simulink library "mylib"  (R2020a)
settings: Solver=VariableStepAuto  StartTime=0.0  StopTime=10.0  RelTol=1e-3
undefined symbols (not defined in the file): d_du_max_pu, dir_to_bus1, dir_to_bus_0L, dir_to_bus_2, dir_to_line1, dir_to_line_0L, dir_to_line_2, du_max_pu, du_ph_max_pu, Fi_0, Fi_T_H, Fi_T_L, Fi_T_M, I0_calc_0L, I0_comp_H, I0_comp_L, I0_comp_M, I0_max_0L, I2_max_2, I_diff1, I_diff2, I_diff3, I_diff4, I_diff5, I_diff_to, I_hight_CT1_G, I_hight_CT2_G, I_low_CT1, I_low_CT2, I_max1, I_max2, I_max3, I_max4, I_max5, I_min_sec_CT1, I_min_sec_CT2, I_unb, Iph_max_0L, Iph_max_2, jmp_in_zone, jmp_in_zone_0L, jmp_in_zone_2, K_dop, max_min1, only_K1_0L, only_K1_2, only_K2_0L, only_K2_2, only_K3_0L, only_K3_2, P_ctl_0, PQ_Fi_ctl_0, Q_ctl_0, S_set_0, set, set1, T_fast, T_I_ctl, T_off, T_on ... (+15)
libraries: $bdroot x184, powerlib_meascontrol x97
(part 2 of 14)

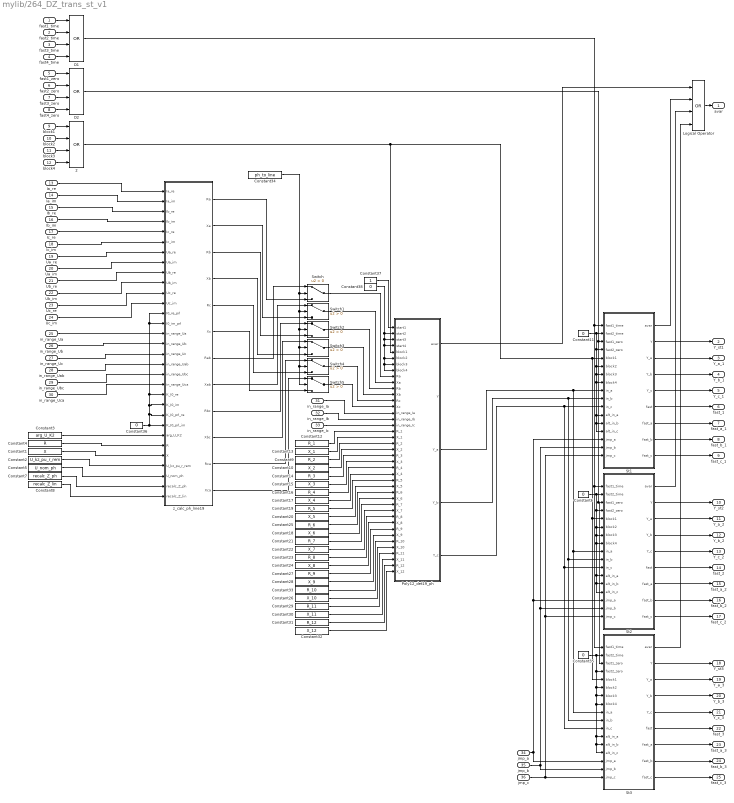
== system mylib/264_DZ_trans_st_v1 ==
  fast1_time : Inport
  fast2_time : Inport  Port=2
  fast3_time : Inport  Port=3
  fast4_time : Inport  Port=4
  fast1_zero : Inport  Port=5
  fast2_zero : Inport  Port=6
  fast3_zero : Inport  Port=7
  fast4_zero : Inport  Port=8
  block1 : Inport  Port=9
  block2 : Inport  Port=10
  block3 : Inport  Port=11
  block4 : Inport  Port=12
  Ia_re : Inport  Port=13
  Ia_im : Inport  Port=14
  Ib_re : Inport  Port=15
  Ib_im : Inport  Port=16
  Ic_re : Inport  Port=17
  Ic_im : Inport  Port=18
  Ua_re : Inport  Port=19
  Ua_im : Inport  Port=20
  Ub_re : Inport  Port=21
  Ub_im : Inport  Port=22
  Uc_re : Inport  Port=23
  Uc_im : Inport  Port=24
  in_range_Ua : Inport  Port=25
  in_range_Ub : Inport  Port=26
  in_range_Uc : Inport  Port=27
  in_range_Uab : Inport  Port=28
  in_range_Ubc : Inport  Port=29
  in_range_Uca : Inport  Port=30
  in_range_Ia : Inport  Port=31
  in_range_Ib : Inport  Port=32
  in_range_Ic : Inport  Port=33
  jmp_a : Inport  Port=34
  jmp_b : Inport  Port=35
  jmp_c : Inport  Port=36
  2 : Logic  Operator=OR  Inputs=4  AllPortsSameDT=off  OutDataTypeStr=boolean
  Constant1 : Constant  Value=X
  Constant10 : Constant  Value=X_2
  Constant{6,11,35..36,38} (5 alike) : Constant  Value=0
  Constant12 : Constant  Value=R_1
  Constant13 : Constant  Value=X_1
  Constant14 : Constant  Value=R_3
  Constant15 : Constant  Value=X_3
  Constant16 : Constant  Value=R_4
  Constant17 : Constant  Value=X_4
  Constant18 : Constant  Value=X_6
  Constant19 : Constant  Value=R_5
  Constant2 : Constant  Value=U_kz_pu_r_rem
  Constant20 : Constant  Value=X_5
  Constant21 : Constant  Value=R_7
  Constant22 : Constant  Value=X_7
  Constant23 : Constant  Value=R_8
  Constant24 : Constant  Value=X_8
  Constant25 : Constant  Value=R_6
  Constant26 : Constant  Value=X_10
  Constant27 : Constant  Value=R_9
  Constant28 : Constant  Value=X_9
  Constant29 : Constant  Value=R_11
  Constant3 : Constant  Value=arg_U_K2
  Constant30 : Constant  Value=X_11
  Constant31 : Constant  Value=R_12
  Constant32 : Constant  Value=X_12
  Constant33 : Constant  Value=R_10
  Constant34 : Constant  Value=ph_to_line
  Constant37 : Constant
  Constant4 : Constant  Value=R
  Constant5 : Constant  Value=U_nom_ph
  Constant7 : Constant  Value=recalc_Z_ph
  Constant8 : Constant  Value=recalc_Z_lin
  Constant9 : Constant  Value=R_2
  D1 : Logic  Operator=OR  Inputs=4  AllPortsSameDT=off  OutDataTypeStr=boolean
  D2 : Logic  Operator=OR  Inputs=4  AllPortsSameDT=off  OutDataTypeStr=boolean
  Logical Operator : Logic  Operator=OR  Inputs=4  AllPortsSameDT=off  OutDataTypeStr=boolean
  Poly12_det19_ph : Subsystem
  St1 : Subsystem  AncestorBlock=mylib/230_st18_ph  mask{st18_ph=[1, 1, 1, jmp_in_zone, T_reset, T_fast, T_st1, T_out]}
      mask prompts: st18_ph "st18_ph [only_K1, only_K2, only_K3, jmp_in_zone, T_reset, T_fast, T_st, T_out]"
      mask init:
      | only_K1 = st18_ph(1);
      | only_K2 = st18_ph(2); 
      | only_K3 = st18_ph(3); 
      | jmp_in_zone = st18_ph(4);
      | T_reset = st18_ph(5);
      | T_fast = st18_ph(6); 
      | T_st = st18_ph(7); 
      | T_out = st18_ph(8);
  St2 : Subsystem  AncestorBlock=mylib/230_st18_ph  mask{st18_ph=[1, 1, 1, jmp_in_zone, T_reset, T_fast, T_st2, T_out]}
      mask prompts: st18_ph "st18_ph [only_K1, only_K2, only_K3, jmp_in_zone, T_reset, T_fast, T_st, T_out]"
      mask init:
      | only_K1 = st18_ph(1);
      | only_K2 = st18_ph(2); 
      | only_K3 = st18_ph(3); 
      | jmp_in_zone = st18_ph(4);
      | T_reset = st18_ph(5);
      | T_fast = st18_ph(6); 
      | T_st = st18_ph(7); 
      | T_out = st18_ph(8);
  St3 : Subsystem  AncestorBlock=mylib/230_st18_ph  mask{st18_ph=[1, 1, 1, jmp_in_zone, T_reset, T_fast, T_st3, T_out]}
      mask prompts: st18_ph "st18_ph [only_K1, only_K2, only_K3, jmp_in_zone, T_reset, T_fast, T_st, T_out]"
      mask init:
      | only_K1 = st18_ph(1);
      | only_K2 = st18_ph(2); 
      | only_K3 = st18_ph(3); 
      | jmp_in_zone = st18_ph(4);
      | T_reset = st18_ph(5);
      | T_fast = st18_ph(6); 
      | T_st = st18_ph(7); 
      | T_out = st18_ph(8);
  Switch{,1..5} (6 alike) : Switch  Criteria=u2 > Threshold
  z_calc_ph_line19 : Subsystem
  avar : Outport
  Y_st1 : Outport  Port=2
  Y_a_1 : Outport  Port=3
  Y_b_1 : Outport  Port=4
  Y_c_1 : Outport  Port=5
  fast_1 : Outport  Port=6
  fast_a_1 : Outport  Port=7
  fast_b_1 : Outport  Port=8
  fast_c_1 : Outport  Port=9
  Y_st2 : Outport  Port=10
  Y_a_2 : Outport  Port=11
  Y_b_2 : Outport  Port=12
  Y_c_2 : Outport  Port=13
  fast_2 : Outport  Port=14
  fast_a_2 : Outport  Port=15
  fast_b_2 : Outport  Port=16
  fast_c_2 : Outport  Port=17
  Y_st3 : Outport  Port=18
  Y_a_3 : Outport  Port=19
  Y_b_3 : Outport  Port=20
  Y_c_3 : Outport  Port=21
  fast_3 : Outport  Port=22
  fast_a_3 : Outport  Port=23
  fast_b_3 : Outport  Port=24
  fast_c_3 : Outport  Port=25
  wires:
  block4/1 -> 2/4
  block3/1 -> 2/3
  block2/1 -> 2/2
  block1/1 -> 2/1
  fast2_time/1 -> D1/2
  fast4_time/1 -> D1/4
  fast3_time/1 -> D1/3
  fast1_time/1 -> D1/1
  St1/2(Y) -> Y_st1/1
  Constant11/1 -> St1/2(fast2_time), St1/14(alt_in_c), St1/13(alt_in_b), St1/12(alt_in_a), St1/8(block4), St1/7(block3), St1/6(block2), St1/4(fast2_zero)
  Logical Operator/1 -> avar/1
  Constant6/1 -> St2/2(fast2_time), St2/14(alt_in_c), St2/13(alt_in_b), St2/12(alt_in_a), St2/8(block4), St2/7(block3), St2/6(block2), St2/4(fast2_zero)
  jmp_a/1 -> St3/15(jmp_a), St1/15(jmp_a), St2/15(jmp_a)
  jmp_c/1 -> St3/17(jmp_c), St1/17(jmp_c), St2/17(jmp_c)
  jmp_b/1 -> St3/16(jmp_b), St1/16(jmp_b), St2/16(jmp_b)
  St2/2(Y) -> Y_st2/1
  St1/1(avar) -> Logical Operator/2
  St2/1(avar) -> Logical Operator/3
  fast3_zero/1 -> D2/3
  fast2_zero/1 -> D2/2
  fast1_zero/1 -> D2/1
  fast4_zero/1 -> D2/4
  Constant35/1 -> St3/2(fast2_time), St3/14(alt_in_c), St3/13(alt_in_b), St3/12(alt_in_a), St3/8(block4), St3/7(block3), St3/6(block2), St3/4(fast2_zero)
  Constant36/1 -> z_calc_ph_line19/23(K_I0_prl_re), z_calc_ph_line19/22(K_I0_im), z_calc_ph_line19/13(I0_re_prl), z_calc_ph_line19/14(I0_im_prl), z_calc_ph_line19/21(K_I0_re), z_calc_ph_line19/24(K_I0_prl_im)
  Ia_re/1 -> z_calc_ph_line19/1(Ia_re)
  Ia_im/1 -> z_calc_ph_line19/2(Ia_im)
  Ib_re/1 -> z_calc_ph_line19/3(Ib_re)
  Ib_im/1 -> z_calc_ph_line19/4(Ib_im)
  Ic_re/1 -> z_calc_ph_line19/5(Ic_re)
  Ic_im/1 -> z_calc_ph_line19/6(Ic_im)
  Ua_re/1 -> z_calc_ph_line19/7(Ua_re)
  Ua_im/1 -> z_calc_ph_line19/8(Ua_im)
  Ub_re/1 -> z_calc_ph_line19/9(Ub_re)
  Ub_im/1 -> z_calc_ph_line19/10(Ub_im)
  Uc_re/1 -> z_calc_ph_line19/11(Uc_re)
  Uc_im/1 -> z_calc_ph_line19/12(Uc_im)
  in_range_Ua/1 -> z_calc_ph_line19/15(in_range_Ua)
  in_range_Ub/1 -> z_calc_ph_line19/16(in_range_Ub)
  in_range_Uc/1 -> z_calc_ph_line19/17(in_range_Uc)
  in_range_Uab/1 -> z_calc_ph_line19/18(in_range_Uab)
  in_range_Ubc/1 -> z_calc_ph_line19/19(in_range_Ubc)
  in_range_Uca/1 -> z_calc_ph_line19/20(in_range_Uca)
  Constant3/1 -> z_calc_ph_line19/25(arg_U_K2)
  Constant4/1 -> z_calc_ph_line19/26(R)
  Constant8/1 -> z_calc_ph_line19/31(recalc_Z_lin)
  Constant7/1 -> z_calc_ph_line19/30(recalc_Z_ph)
  Constant5/1 -> z_calc_ph_line19/29(U_nom_ph)
  Constant2/1 -> z_calc_ph_line19/28(U_kz_pu_r_rem)
  Constant1/1 -> z_calc_ph_line19/27(X)
  Constant12/1 -> Poly12_det19_ph/18(R_1)
  Constant13/1 -> Poly12_det19_ph/19(X_1)
  Constant9/1 -> Poly12_det19_ph/20(R_2)
  Constant10/1 -> Poly12_det19_ph/21(X_2)
  Constant32/1 -> Poly12_det19_ph/41(X_12)
  Constant31/1 -> Poly12_det19_ph/40(R_12)
  Constant30/1 -> Poly12_det19_ph/39(X_11)
  Constant29/1 -> Poly12_det19_ph/38(R_11)
  Constant26/1 -> Poly12_det19_ph/37(X_10)
  Constant33/1 -> Poly12_det19_ph/36(R_10)
  Constant28/1 -> Poly12_det19_ph/35(X_9)
  Constant27/1 -> Poly12_det19_ph/34(R_9)
  Constant24/1 -> Poly12_det19_ph/33(X_8)
  Constant23/1 -> Poly12_det19_ph/32(R_8)
  Constant22/1 -> Poly12_det19_ph/31(X_7)
  Constant21/1 -> Poly12_det19_ph/30(R_7)
  Constant18/1 -> Poly12_det19_ph/29(X_6)
  Constant25/1 -> Poly12_det19_ph/28(R_6)
  Constant20/1 -> Poly12_det19_ph/27(X_5)
  Constant19/1 -> Poly12_det19_ph/26(R_5)
  Constant17/1 -> Poly12_det19_ph/25(X_4)
  Constant16/1 -> Poly12_det19_ph/24(R_4)
  Constant15/1 -> Poly12_det19_ph/23(X_3)
  Constant14/1 -> Poly12_det19_ph/22(R_3)
  Constant34/1 -> Switch5/2, Switch4/2, Switch3/2, Switch2/2, Switch1/2, Switch/2
  z_calc_ph_line19/7(Rab) -> Switch/1
  z_calc_ph_line19/8(Xab) -> Switch1/1
  z_calc_ph_line19/9(Rbc) -> Switch2/1
  z_calc_ph_line19/10(Xbc) -> Switch3/1
  z_calc_ph_line19/11(Rca) -> Switch4/1
  z_calc_ph_line19/12(Xca) -> Switch5/1
  z_calc_ph_line19/6(Xc) -> Switch5/3
  z_calc_ph_line19/5(Rc) -> Switch4/3
  z_calc_ph_line19/4(Xb) -> Switch3/3
  z_calc_ph_line19/3(Rb) -> Switch2/3
  z_calc_ph_line19/2(Xa) -> Switch1/3
  z_calc_ph_line19/1(Ra) -> Switch/3
  Switch5/1 -> Poly12_det19_ph/14(Xc)
  Switch4/1 -> Poly12_det19_ph/13(Rc)
  Switch3/1 -> Poly12_det19_ph/12(Xb)
  Switch2/1 -> Poly12_det19_ph/11(Rb)
  Switch1/1 -> Poly12_det19_ph/10(Xa)
  Switch/1 -> Poly12_det19_ph/9(Ra)
  in_range_Ic/1 -> Poly12_det19_ph/17(in_range_Ic)
  in_range_Ib/1 -> Poly12_det19_ph/16(in_range_Ib)
  in_range_Ia/1 -> Poly12_det19_ph/15(in_range_Ia)
  Poly12_det19_ph/3(Y_a) -> St3/9(in_a), St2/9(in_a), St1/9(in_a)
  Poly12_det19_ph/4(Y_b) -> St3/10(in_b), St2/10(in_b), St1/10(in_b)
  Poly12_det19_ph/5(Y_c) -> St3/11(in_c), St2/11(in_c), St1/11(in_c)
  St3/2(Y) -> Y_st3/1
  Poly12_det19_ph/1(avar) -> Logical Operator/1
  St3/1(avar) -> Logical Operator/4
  St1/3(Y_a) -> Y_a_1/1
  St1/4(Y_b) -> Y_b_1/1
  St1/5(Y_c) -> Y_c_1/1
  St1/6(fast) -> fast_1/1
  St1/7(fast_a) -> fast_a_1/1
  St1/9(fast_c) -> fast_c_1/1
  St1/8(fast_b) -> fast_b_1/1
  St2/3(Y_a) -> Y_a_2/1
  St2/4(Y_b) -> Y_b_2/1
  St2/5(Y_c) -> Y_c_2/1
  St2/6(fast) -> fast_2/1
  St2/7(fast_a) -> fast_a_2/1
  St2/8(fast_b) -> fast_b_2/1
  St2/9(fast_c) -> fast_c_2/1
  St3/9(fast_c) -> fast_c_3/1
  St3/8(fast_b) -> fast_b_3/1
  St3/7(fast_a) -> fast_a_3/1
  St3/6(fast) -> fast_3/1
  St3/5(Y_c) -> Y_c_3/1
  St3/4(Y_b) -> Y_b_3/1
  St3/3(Y_a) -> Y_a_3/1
  2/1 -> Poly12_det19_ph/5(block1), St3/5(block1), St2/5(block1), St1/5(block1)
  Constant37/1 -> Poly12_det19_ph/1(start1)
  Constant38/1 -> Poly12_det19_ph/8(block4), Poly12_det19_ph/7(block3), Poly12_det19_ph/6(block2), Poly12_det19_ph/4(start4), Poly12_det19_ph/3(start3), Poly12_det19_ph/2(start2)
  D2/1 -> St3/3(fast1_zero), St2/3(fast1_zero), St1/3(fast1_zero)
  D1/1 -> St3/1(fast1_time), St2/1(fast1_time), St1/1(fast1_time)

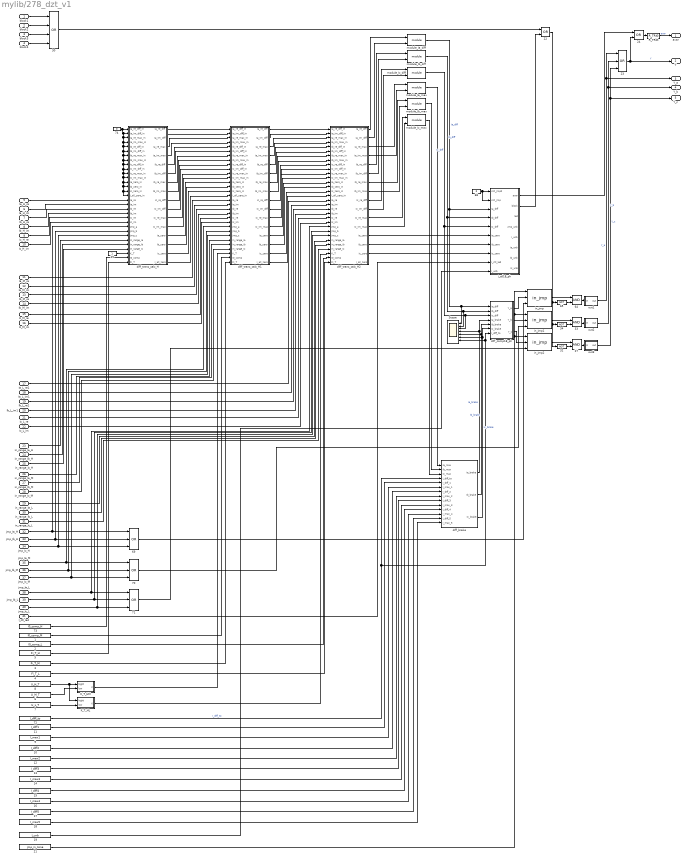
== system mylib/278_dzt_v1 ==
  block1 : Inport
  block2 : Inport  Port=2
  block3 : Inport  Port=3
  block4 : Inport  Port=4
  Ia_H_re : Inport  Port=5
  Ia_H_im : Inport  Port=6
  Ib_H_re : Inport  Port=7
  Ib_H_im : Inport  Port=8
  Ic_H_re : Inport  Port=9
  Ic_H_im : Inport  Port=10
  Ia_M_re : Inport  Port=11
  Ia_M_im : Inport  Port=12
  Ib_M_re : Inport  Port=13
  Ib_M_im : Inport  Port=14
  Ic_M_re : Inport  Port=15
  Ic_M_im : Inport  Port=16
  Ia_L_re1 : Inport  Port=17
  Ia_L_im1 : Inport  Port=18
  Ib_L_re1 : Inport  Port=19
  Ib_L_im1 : Inport  Port=20
  Ic_L_re : Inport  Port=21
  Ic_L_im : Inport  Port=22
  in_range_Ia_H : Inport  Port=23
  in_range_Ib_H : Inport  Port=24
  in_range_Ic_H : Inport  Port=25
  in_range_Ia_M : Inport  Port=26
  in_range_Ib_M : Inport  Port=27
  in_range_Ic_M : Inport  Port=28
  in_range_Ia_L : Inport  Port=29
  in_range_Ib_L : Inport  Port=30
  in_range_Ic_L : Inport  Port=31
  jmp_Ia_H : Inport  Port=32
  jmp_Ib_H : Inport  Port=33
  jmp_Ic_H : Inport  Port=34
  jmp_Ia_M : Inport  Port=35
  jmp_Ib_M : Inport  Port=36
  jmp_Ic_M : Inport  Port=37
  jmp_Ia_L : Inport  Port=38
  jmp_Ib_L : Inport  Port=39
  jmp_Ic_L : Inport  Port=40
  I_ctl_led : Inport  Port=41
  1 : Constant  Value=I0_comp_M
  10 : Constant  Value=I_diff2
  11 : Constant  Value=I_diff1
  12 : Constant  Value=I_max2
  13 : Constant  Value=I_diff3
  14 : Constant  Value=I_max3
  15 : Constant  Value=I_diff4
  16 : Constant  Value=I_max4
  17 : Constant  Value=I_diff5
  18 : Constant  Value=I_max5
  19 : Constant  Value=I_unb
  2 : Constant  Value=I0_comp_L
  21 : Constant  Value=jmp_in_zone
  22 : Logic  Operator=OR  AllPortsSameDT=off  OutDataTypeStr=boolean
  {23,69..71} (4 alike) : Logic  Operator=OR  Inputs=3  AllPortsSameDT=off  OutDataTypeStr=boolean
  24 : Logic  Operator=OR  AllPortsSameDT=off  OutDataTypeStr=boolean
  25 : Constant
  27 : Logic  AllPortsSameDT=off  OutDataTypeStr=boolean
  3 : Constant  Value=Fi_T_M
  30 : Logic  Operator=OR  Inputs=4  AllPortsSameDT=off  OutDataTypeStr=boolean
  32 : Logic  Operator=NOT  AllPortsSameDT=off  OutDataTypeStr=boolean
  33 : Logic  AllPortsSameDT=off  OutDataTypeStr=boolean
  34 : Logic  Operator=NOT  AllPortsSameDT=off  OutDataTypeStr=boolean
  4 : Constant  Value=Fi_T_L
  5 : Constant  Value=Fi_T_H
  6 : Constant  Value=U_M_T
  64 : Logic  AllPortsSameDT=off  OutDataTypeStr=boolean
  65 : Logic  Operator=NOT  AllPortsSameDT=off  OutDataTypeStr=boolean
  68 : Constant  Value=0
  7 : Constant  Value=U_L_T
  72 : Constant  Value=I_diff_to
  73 : Constant  Value=I0_comp_H
  74 : Constant  Value=0
  8 : Constant  Value=U_H_T
  9 : Constant  Value=I_max1
  K_T_HL : Subsystem
  K_T_HM : Subsystem
  R_TRIG : $bdroot/R_TRIG  SystemSampleTime=-1  Latency=0  AutoFrameSizeCalculation=off
  Scope : Scope  NumInputPorts=7
  diff_brake : Subsystem
  diff_comp18_ph : Subsystem
  diff_trans_calc_H : Subsystem
  diff_trans_calc_H1 : Subsystem
  diff_trans_calc_H2 : Subsystem
  i_ctl18_ph : Subsystem  mask{CTL=[T_I_ctl]}
      mask prompts: CTL "CTL[T_I_ctl]"
      mask init:
      | T_I_ctl = CTL(1);
  in_jmp : $bdroot/in_jmp  in_jmp=[T_reset]
  in_jmp1 : $bdroot/in_jmp  in_jmp=[T_reset]
  in_jmp2 : $bdroot/in_jmp  in_jmp=[T_reset]
  module_Ia_diff : $bdroot/module  SystemSampleTime=-1  Latency=0  AutoFrameSizeCalculation=off
  module_Ia_max : $bdroot/module  SystemSampleTime=-1  Latency=0  AutoFrameSizeCalculation=off
  module_Ib_diff : $bdroot/module  SystemSampleTime=-1  Latency=0  AutoFrameSizeCalculation=off
  module_Ib_max : $bdroot/module  SystemSampleTime=-1  Latency=0  AutoFrameSizeCalculation=off
  module_Ic_diff : $bdroot/module  SystemSampleTime=-1  Latency=0  AutoFrameSizeCalculation=off
  module_Ic_max : $bdroot/module  SystemSampleTime=-1  Latency=0  AutoFrameSizeCalculation=off
  out1 : Subsystem  mask{out=[T_out]}
      mask prompts: out "out[T_out]"
      mask init:
      | T_out = out(1);
  out2 : Subsystem  mask{out=[T_out]}
      mask prompts: out "out[T_out]"
      mask init:
      | T_out = out(1);
  out3 : Subsystem  mask{out=[T_out]}
      mask prompts: out "out[T_out]"
      mask init:
      | T_out = out(1);
  avar : Outport
  Y : Outport  Port=2
  Y_a : Outport  Port=3
  Y_b : Outport  Port=4
  Y_c : Outport  Port=5
  wires:
  I_ctl_led/1 -> i_ctl18_ph/9(I_ctl_led)
  22/1 -> 65/1, 34/1, 32/1
  R_TRIG/1 -> avar/1  "avar"
  out3/1(out) -> 23/3, Y_c/1  "Y_c"
  out2/1(out) -> 23/2, Y_b/1  "Y_b"
  out1/1(out) -> 23/1, Y_a/1  "Y_a"
  i_ctl18_ph/1(avar) -> 24/1
  24/1 -> R_TRIG/1
  23/1 -> Y/1, 24/2  "Y"
  30/1 -> 22/1
  i_ctl18_ph/2(block) -> 22/2
  65/1 -> 64/2
  34/1 -> 33/2
  in_range_Ib_M/1 -> diff_trans_calc_H1/27(in_range_Ib)
  jmp_Ic_L/1 -> 71/3, diff_trans_calc_H2/25(jmp_c)
  in_range_Ic_L/1 -> diff_trans_calc_H2/28(in_range_Ic)
  jmp_Ia_L/1 -> 71/1, diff_trans_calc_H2/23(jmp_a)
  jmp_Ib_M/1 -> 70/2, diff_trans_calc_H1/24(jmp_b)
  jmp_Ia_M/1 -> 70/1, diff_trans_calc_H1/23(jmp_a)
  jmp_Ib_H/1 -> 69/2, diff_trans_calc_H/24(jmp_b)
  jmp_Ic_H/1 -> 69/3, diff_trans_calc_H/25(jmp_c)
  in_range_Ib_H/1 -> diff_trans_calc_H/27(in_range_Ib)
  in_range_Ic_H/1 -> diff_trans_calc_H/28(in_range_Ic)
  in_range_Ia_L/1 -> diff_trans_calc_H2/26(in_range_Ia)
  jmp_Ia_H/1 -> diff_trans_calc_H/23(jmp_a), 69/1
  74/1 -> diff_trans_calc_H/1(Ia_re_diff_in), diff_trans_calc_H/2(Ia_im_diff_in), diff_trans_calc_H/16(I_all_zero_in), diff_trans_calc_H/15(Ic_zero_in), diff_trans_calc_H/14(Ib_zero_in), diff_trans_calc_H/13(Ia_zero_in), diff_trans_calc_H/12(Ic_im_max_in), diff_trans_calc_H/11(Ic_re_max_in), diff_trans_calc_H/10(Ic_im_diff_in), diff_trans_calc_H/9(Ic_re_diff_in), diff_trans_calc_H/8(Ib_im_max_in), diff_trans_calc_H/7(Ib_re_max_in), diff_trans_calc_H/6(Ib_im_diff_in), diff_trans_calc_H/5(Ib_re_diff_in), diff_trans_calc_H/4(Ia_im_max_in), diff_trans_calc_H/3(Ia_re_max_in)
  73/1 -> diff_trans_calc_H/30(I0_comp)
  Ic_L_re/1 -> diff_trans_calc_H2/21(Ic_re)
  Ib_L_im1/1 -> diff_trans_calc_H2/20(Ib_im)
  Ib_L_re1/1 -> diff_trans_calc_H2/19(Ib_re)
  Ia_L_im1/1 -> diff_trans_calc_H2/18(Ia_im)
  Ic_L_im/1 -> diff_trans_calc_H2/22(Ic_im)
  Ia_L_re1/1 -> diff_trans_calc_H2/17(Ia_re)
  diff_trans_calc_H1/2(Ia_im_diff) -> diff_trans_calc_H2/2(Ia_im_diff_in)
  diff_trans_calc_H1/3(Ia_re_max) -> diff_trans_calc_H2/3(Ia_re_max_in)
  diff_trans_calc_H1/4(Ia_im_max) -> diff_trans_calc_H2/4(Ia_im_max_in)
  diff_trans_calc_H1/5(Ib_re_diff) -> diff_trans_calc_H2/5(Ib_re_diff_in)
  diff_trans_calc_H1/6(Ib_im_diff) -> diff_trans_calc_H2/6(Ib_im_diff_in)
  diff_trans_calc_H1/7(Ib_re_max) -> diff_trans_calc_H2/7(Ib_re_max_in)
  diff_trans_calc_H1/8(Ib_im_max) -> diff_trans_calc_H2/8(Ib_im_max_in)
  diff_trans_calc_H1/9(Ic_re_diff) -> diff_trans_calc_H2/9(Ic_re_diff_in)
  diff_trans_calc_H1/10(Ic_im_diff) -> diff_trans_calc_H2/10(Ic_im_diff_in)
  diff_trans_calc_H1/11(Ic_re_max) -> diff_trans_calc_H2/11(Ic_re_max_in)
  diff_trans_calc_H1/12(Ic_im_max) -> diff_trans_calc_H2/12(Ic_im_max_in)
  diff_trans_calc_H1/13(Ia_zero) -> diff_trans_calc_H2/13(Ia_zero_in)
  diff_trans_calc_H1/14(Ib_zero) -> diff_trans_calc_H2/14(Ib_zero_in)
  diff_trans_calc_H1/15(Ic_zero) -> diff_trans_calc_H2/15(Ic_zero_in)
  2/1 -> diff_trans_calc_H2/30(I0_comp)
  4/1 -> diff_trans_calc_H2/31(Fi_T)
  K_T_HL/1(K) -> diff_trans_calc_H2/29(K_T)
  K_T_HM/1(K) -> diff_trans_calc_H1/29(K_T)
  3/1 -> diff_trans_calc_H1/31(Fi_T)
  diff_trans_calc_H/2(Ia_im_diff) -> diff_trans_calc_H1/2(Ia_im_diff_in)
  diff_trans_calc_H/3(Ia_re_max) -> diff_trans_calc_H1/3(Ia_re_max_in)
  diff_trans_calc_H/4(Ia_im_max) -> diff_trans_calc_H1/4(Ia_im_max_in)
  diff_trans_calc_H/5(Ib_re_diff) -> diff_trans_calc_H1/5(Ib_re_diff_in)
  diff_trans_calc_H/6(Ib_im_diff) -> diff_trans_calc_H1/6(Ib_im_diff_in)
  diff_trans_calc_H/7(Ib_re_max) -> diff_trans_calc_H1/7(Ib_re_max_in)
  diff_trans_calc_H/8(Ib_im_max) -> diff_trans_calc_H1/8(Ib_im_max_in)
  diff_trans_calc_H/9(Ic_re_diff) -> diff_trans_calc_H1/9(Ic_re_diff_in)
  diff_trans_calc_H/10(Ic_im_diff) -> diff_trans_calc_H1/10(Ic_im_diff_in)
  diff_trans_calc_H/11(Ic_re_max) -> diff_trans_calc_H1/11(Ic_re_max_in)
  diff_trans_calc_H/12(Ic_im_max) -> diff_trans_calc_H1/12(Ic_im_max_in)
  diff_trans_calc_H/13(Ia_zero) -> diff_trans_calc_H1/13(Ia_zero_in)
  diff_trans_calc_H/14(Ib_zero) -> diff_trans_calc_H1/14(Ib_zero_in)
  diff_trans_calc_H/15(Ic_zero) -> diff_trans_calc_H1/15(Ic_zero_in)
  Ib_M_re/1 -> diff_trans_calc_H1/19(Ib_re)
  Ib_M_im/1 -> diff_trans_calc_H1/20(Ib_im)
  Ic_M_re/1 -> diff_trans_calc_H1/21(Ic_re)
  Ic_M_im/1 -> diff_trans_calc_H1/22(Ic_im)
  Ia_M_im/1 -> diff_trans_calc_H1/18(Ia_im)
  Ia_M_re/1 -> diff_trans_calc_H1/17(Ia_re)
  Ic_H_re/1 -> diff_trans_calc_H/21(Ic_re)
  Ic_H_im/1 -> diff_trans_calc_H/22(Ic_im)
  Ib_H_im/1 -> diff_trans_calc_H/20(Ib_im)
  Ib_H_re/1 -> diff_trans_calc_H/19(Ib_re)
  Ia_H_im/1 -> diff_trans_calc_H/18(Ia_im)
  Ia_H_re/1 -> diff_trans_calc_H/17(Ia_re)
  module_Ic_max/1 -> diff_brake/3(Ic_max)
  module_Ib_max/1 -> diff_brake/2(Ib_max)
  module_Ia_max/1 -> diff_brake/1(Ia_max)
  18/1 -> diff_brake/14(I_max_5)
  17/1 -> diff_brake/13(I_diff_5)
  16/1 -> diff_brake/12(I_max_4)
  15/1 -> diff_brake/11(I_diff_4)
  14/1 -> diff_brake/10(I_max_3)
  13/1 -> diff_brake/9(I_diff_3)
  12/1 -> diff_brake/8(I_max_2)
  10/1 -> diff_brake/7(I_diff_2)
  9/1 -> diff_brake/6(I_max_1)
  11/1 -> diff_brake/5(I_diff_1)
  72/1 -> diff_comp18_ph/7(I_diff_to), Scope/7, diff_brake/4(I_diff_to)  "I_diff_to"
  69/1 -> in_jmp/3
  70/1 -> in_jmp1/3
  71/1 -> in_jmp2/3
  jmp_Ic_M/1 -> 70/3, diff_trans_calc_H1/25(jmp_c)
  jmp_Ib_L/1 -> 71/2, diff_trans_calc_H2/24(jmp_b)
  21/1 -> in_jmp/1, in_jmp1/1, in_jmp2/1
  module_Ib_diff/1 -> i_ctl18_ph/4(Ib_diff), diff_comp18_ph/2(Ib_diff), Scope/2  "Ib_diff"
  68/1 -> i_ctl18_ph/1(cnt_jmp0), i_ctl18_ph/2(cnt_jmp)
  diff_trans_calc_H2/15(Ic_zero) -> i_ctl18_ph/8(Ic_zero)
  diff_trans_calc_H2/14(Ib_zero) -> i_ctl18_ph/7(Ib_zero)
  diff_trans_calc_H2/13(Ia_zero) -> i_ctl18_ph/6(Ia_zero)
  module_Ia_diff/1 -> i_ctl18_ph/3(Ia_diff), diff_comp18_ph/1(Ia_diff), Scope/1  "Ia_diff"
  module_Ic_diff/1 -> i_ctl18_ph/5(Ic_diff), diff_comp18_ph/3(Ic_diff), Scope/3  "Ic_diff"
  diff_comp18_ph/1(Y_a) -> in_jmp/2
  diff_comp18_ph/2(Y_b) -> in_jmp1/2
  diff_comp18_ph/3(Y_c) -> in_jmp2/2
  diff_trans_calc_H2/1(Ia_re_diff) -> module_Ia_diff/1
  diff_trans_calc_H2/2(Ia_im_diff) -> module_Ia_diff/2
  diff_trans_calc_H2/9(Ic_re_diff) -> module_Ic_diff/1
  diff_trans_calc_H2/3(Ia_re_max) -> module_Ia_max/1
  diff_trans_calc_H2/4(Ia_im_max) -> module_Ia_max/2
  diff_trans_calc_H2/10(Ic_im_diff) -> module_Ic_diff/2
  diff_trans_calc_H2/5(Ib_re_diff) -> module_Ib_diff/1
  diff_trans_calc_H2/6(Ib_im_diff) -> module_Ib_diff/2
  diff_trans_calc_H2/7(Ib_re_max) -> module_Ib_max/1
  diff_trans_calc_H2/8(Ib_im_max) -> module_Ib_max/2
  diff_trans_calc_H2/12(Ic_im_max) -> module_Ic_max/2
  diff_trans_calc_H2/11(Ic_re_max) -> module_Ic_max/1
  diff_brake/3(Ic_brake) -> diff_comp18_ph/6(Ic_brake), Scope/6  "Ic_brake"
  diff_brake/2(Ib_brake) -> Scope/5, diff_comp18_ph/5(Ib_brake)  "Ib_brake"
  diff_brake/1(Ia_brake) -> Scope/4, diff_comp18_ph/4(Ia_brake)  "Ia_brake"
  27/1 -> out3/1(in)
  33/1 -> out2/1(in)
  64/1 -> out1/1(in)
  in_jmp/1 -> 64/1
  in_jmp1/1 -> 33/1
  in_jmp2/1 -> 27/1
  32/1 -> 27/2
  19/1 -> i_ctl18_ph/10("I_unb ")
  diff_trans_calc_H1/1(Ia_re_diff) -> diff_trans_calc_H2/1(Ia_re_diff_in)
  diff_trans_calc_H1/16(I_all_zero) -> diff_trans_calc_H2/16(I_all_zero_in)
  diff_trans_calc_H/1(Ia_re_diff) -> diff_trans_calc_H1/1(Ia_re_diff_in)
  diff_trans_calc_H/16(I_all_zero) -> diff_trans_calc_H1/16(I_all_zero_in)
  25/1 -> diff_trans_calc_H/29(K_T)
  1/1 -> diff_trans_calc_H1/30(I0_comp)
  5/1 -> diff_trans_calc_H/31(Fi_T)
  in_range_Ic_M/1 -> diff_trans_calc_H1/28(in_range_Ic)
  in_range_Ib_L/1 -> diff_trans_calc_H2/27(in_range_Ib)
  in_range_Ia_M/1 -> diff_trans_calc_H1/26(in_range_Ia)
  in_range_Ia_H/1 -> diff_trans_calc_H/26(in_range_Ia)
  7/1 -> K_T_HL/2(low)
  6/1 -> K_T_HM/2(low)
  8/1 -> K_T_HM/1(hight), K_T_HL/1(hight)
  block1/1 -> 30/1
  block2/1 -> 30/2
  block3/1 -> 30/3
  block4/1 -> 30/4

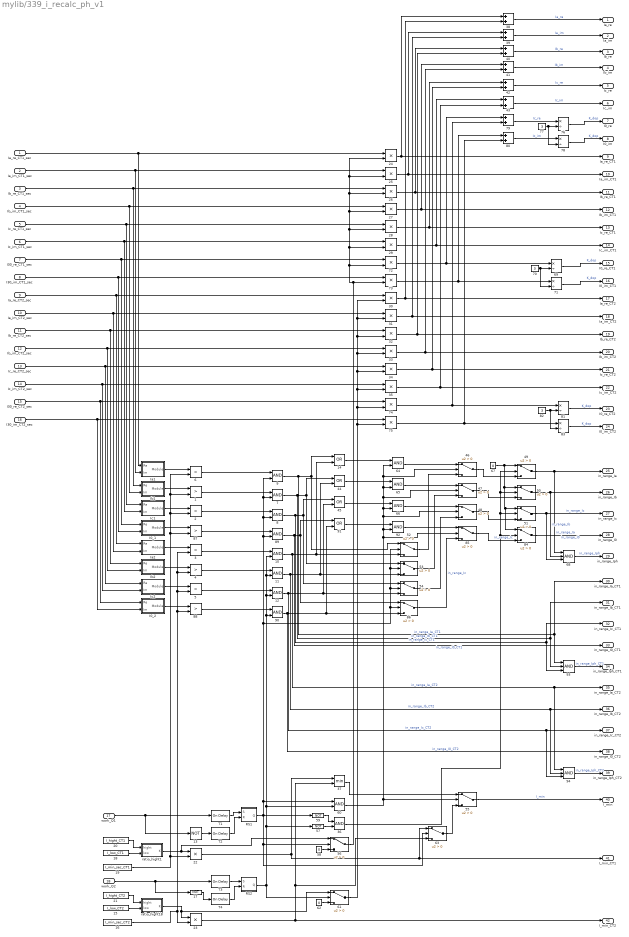
== system mylib/339_i_recalc_ph_v1 ==
  Ia_re_CT1_sec : Inport
  Ia_im_CT1_sec : Inport  Port=2
  Ib_re_CT1_sec : Inport  Port=3
  Ib_im_CT1_sec : Inport  Port=4
  Ic_re_CT1_sec : Inport  Port=5
  Ic_im_CT1_sec : Inport  Port=6
  I30_re_CT1_sec : Inport  Port=7
  I30_im_CT1_sec : Inport  Port=8
  Ia_re_CT2_sec : Inport  Port=9
  Ia_im_CT2_sec : Inport  Port=10
  Ib_re_CT2_sec : Inport  Port=11
  Ib_im_CT2_sec : Inport  Port=12
  Ic_re_CT2_sec : Inport  Port=13
  Ic_im_CT2_sec : Inport  Port=14
  I30_re_CT2_sec : Inport  Port=15
  I30_im_CT2_sec : Inport  Port=16
  work_Q1 : Inport  Port=17
  work_Q2 : Inport  Port=18
  {1..6,87..88} (8 alike) : RelationalOperator  Operator=>  OutDataTypeStr=boolean  RndMeth=Nearest
  {7..12,36,60,64..66,89..90,92} (14 alike) : Logic  AllPortsSameDT=off  OutDataTypeStr=boolean
  {13,17,57,59} (4 alike) : Logic  Operator=NOT  AllPortsSameDT=off  OutDataTypeStr=boolean
  {14,44..45,91} (4 alike) : Logic  Operator=OR  AllPortsSameDT=off  OutDataTypeStr=boolean
  15 : Constant  Value=I_low_CT2
  16 : Constant  Value=I_min_sec_CT2
  18 : Constant  Value=I_low_CT1
  19 : Constant  Value=I_min_sec_CT1
  20 : Constant  Value=I_hight_CT1
  21 : Constant  Value=I_hight_CT2
  {22..35,72..75} (18 alike) : Product  Inputs=**  RndMeth=Zero  SaturateOnIntegerOverflow=on
  37 : MinMax  Inputs=2
  {38..43,79..80} (8 alike) : Sum
  {46..56,61,63,84..86} (16 alike) : Switch  Criteria=u2 > Threshold
  58 : Constant  Value=0
  62 : Constant  Value=0
  67 : Constant  Value=0
  68 : Logic  Inputs=3  AllPortsSameDT=off  OutDataTypeStr=boolean
  {69,71,76,78,81,83} (6 alike) : Product  Inputs=*/  RndMeth=Zero  SaturateOnIntegerOverflow=on
  70 : Constant  Value=3
  77 : Constant  Value=3
  82 : Constant  Value=3
  93 : Logic  Inputs=3  AllPortsSameDT=off  OutDataTypeStr=boolean
  94 : Logic  Inputs=3  AllPortsSameDT=off  OutDataTypeStr=boolean
  I0_1 : Subsystem
  I0_2 : Subsystem
  Ia1 : Subsystem
  Ia2 : Subsystem
  Ib1 : Subsystem
  Ib2 : Subsystem
  Ic1 : Subsystem
  Ic2 : Subsystem
  RS1 : Subsystem
  RS2 : Subsystem
  T1 : powerlib_meascontrol/Logic/On Delay  DelayType=On delay  delay=T_on  ic=0  Ts=0
  T2 : powerlib_meascontrol/Logic/On Delay  DelayType=On delay  delay=T_off  ic=0  Ts=0
  T3 : powerlib_meascontrol/Logic/On Delay  DelayType=On delay  delay=T_on  ic=0  Ts=0
  T4 : powerlib_meascontrol/Logic/On Delay  DelayType=On delay  delay=T_off  ic=0  Ts=0
  ratio_hight1 : Subsystem
  ratio_hight18 : Subsystem
  Ia_re : Outport
  Ia_im : Outport  Port=2
  Ib_re : Outport  Port=3
  Ib_im : Outport  Port=4
  Ic_re : Outport  Port=5
  Ic_im : Outport  Port=6
  I0_re : Outport  Port=7
  I0_im : Outport  Port=8
  Ia_re_CT1 : Outport  Port=9
  Ia_im_CT1 : Outport  Port=10
  Ib_re_CT1 : Outport  Port=11
  Ib_im_CT1 : Outport  Port=12
  Ic_re_CT1 : Outport  Port=13
  Ic_im_CT1 : Outport  Port=14
  I0_re_CT1 : Outport  Port=15
  I0_im_CT1 : Outport  Port=16
  Ia_re_CT2 : Outport  Port=17
  Ia_im_CT2 : Outport  Port=18
  Ib_re_CT2 : Outport  Port=19
  Ib_im_CT2 : Outport  Port=20
  Ic_re_CT2 : Outport  Port=21
  Ic_im_CT2 : Outport  Port=22
  I0_re_CT2 : Outport  Port=23
  I0_im_CT2 : Outport  Port=24
  in_range_Ia : Outport  Port=25
  in_range_Ib : Outport  Port=26
  in_range_Ic : Outport  Port=27
  in_range_I0 : Outport  Port=28
  in_range_Iph : Outport  Port=29
  in_range_Ia_CT1 : Outport  Port=30
  in_range_Ib_CT1 : Outport  Port=31
  in_range_Ic_CT1 : Outport  Port=32
  in_range_I0_CT1 : Outport  Port=33
  in_range_Iph_CT1 : Outport  Port=34
  in_range_Ia_CT2 : Outport  Port=35
  in_range_Ib_CT2 : Outport  Port=36
  in_range_Ic_CT2 : Outport  Port=37
  in_range_I0_CT2 : Outport  Port=38
  in_range_Iph_CT2 : Outport  Port=39
  I_min : Outport  Port=40
  I_min_CT1 : Outport  Port=41
  I_min_CT2 : Outport  Port=42
  wires:
  4/1 -> 11/1
  Ib1/1(Module) -> 1/1
  Ib2/1(Module) -> 4/1
  Ic2/1(Module) -> 5/1
  Ic1/1(Module) -> 2/1
  2/1 -> 8/1
  Ia1/1(Module) -> 6/1
  Ia_re_CT1_sec/1 -> Ia1/1(Re), 24/1
  Ib_im_CT2_sec/1 -> 33/1, Ib2/2(Im)
  Ib_im_CT1_sec/1 -> Ib1/2(Im), 27/1
  Ib_re_CT2_sec/1 -> 32/1, Ib2/1(Re)
  Ia_re_CT2_sec/1 -> 30/1, Ia2/1(Re)
  23/1 -> I_min_CT2/1, 37/2, 63/3
  Ib_re_CT1_sec/1 -> Ib1/1(Re), 26/1
  Ia_im_CT2_sec/1 -> 31/1, Ia2/2(Im)
  13/1 -> T2/1
  RS1/1(Q) -> 59/1, 60/1, 52/2, 53/2, 54/2, 86/2, 89/2, 7/2, 9/2, 8/2, 56/2, 63/2
  Ic_re_CT2_sec/1 -> 34/1, Ic2/1(Re)
  T1/1 -> RS1/1(S)
  Ic_im_CT2_sec/1 -> 35/1, Ic2/2(Im)
  T2/1 -> RS1/2(R)
  19/1 -> 87/2, 2/2, 1/2, 6/2, 22/2
  Ic_re_CT1_sec/1 -> Ic1/1(Re), 28/1
  16/1 -> 23/2, 88/2, 5/2, 4/2, 3/2
  Ic_im_CT1_sec/1 -> Ic1/2(Im), 29/1
  6/1 -> 9/1
  20/1 -> ratio_hight1/1(hight)
  18/1 -> ratio_hight1/2(low)
  ratio_hight1/1(K) -> 56/1, 22/1
  15/1 -> ratio_hight18/2(low)
  ratio_hight18/1(K) -> 61/1, 23/1
  21/1 -> ratio_hight18/1(hight)
  Ia2/1(Module) -> 3/1
  5/1 -> 12/1
  3/1 -> 10/1
  1/1 -> 7/1
  Ia_im_CT1_sec/1 -> Ia1/2(Im), 25/1
  17/1 -> T4/1
  T3/1 -> RS2/1(S)
  T4/1 -> RS2/2(R)
  work_Q1/1 -> 13/1, T1/1
  work_Q2/1 -> 17/1, T3/1
  24/1 -> Ia_re_CT1/1, 38/1
  30/1 -> Ia_re_CT2/1, 38/2
  26/1 -> Ib_re_CT1/1, 40/1
  32/1 -> Ib_re_CT2/1, 40/2
  27/1 -> Ib_im_CT1/1, 41/1
  33/1 -> Ib_im_CT2/1, 41/2
  28/1 -> Ic_re_CT1/1, 42/1
  34/1 -> Ic_re_CT2/1, 42/2
  29/1 -> Ic_im_CT1/1, 43/1
  35/1 -> Ic_im_CT2/1, 43/2
  38/1 -> Ia_re/1  "Ia_re"
  39/1 -> Ia_im/1  "Ia_im"
  40/1 -> Ib_re/1  "Ib_re"
  41/1 -> Ib_im/1  "Ib_im"
  42/1 -> Ic_re/1  "Ic_re"
  43/1 -> Ic_im/1  "Ic_im"
  57/1 -> 36/2
  59/1 -> 36/1
  22/1 -> 37/1, 63/1, I_min_CT1/1
  58/1 -> 56/3
  RS2/1(Q) -> 61/2, 57/1, 60/2, 90/2, 10/2, 11/2, 12/2
  62/1 -> 61/3
  63/1 -> 55/3
  37/1 -> 55/1
  60/1 -> 64/2, 46/2, 65/2, 47/2, 66/2, 48/2, 92/2, 85/2, 55/2
  64/1 -> 46/1
  65/1 -> 47/1
  66/1 -> 48/1
  54/1 -> 48/3
  53/1 -> 47/3
  52/1 -> 46/3
  56/1 -> 72/2, 29/2, 24/2, 25/2, 26/2, 27/2, 28/2, 73/2
  67/1 -> 84/1, 51/1, 50/1, 49/1
  46/1 -> 49/3
  47/1 -> 50/3
  48/1 -> 51/3
  36/1 -> 84/2, 49/2, 50/2, 51/2
  49/1 -> 68/1, in_range_Ia/1  "in_range_Ia"
  51/1 -> 68/3, in_range_Ic/1  "in_range_Ic"
  55/1 -> I_min/1  "I_min"
  14/1 -> 64/1
  44/1 -> 65/1
  45/1 -> 66/1
  61/1 -> 74/2, 35/2, 34/2, 30/2, 31/2, 32/2, 33/2, 75/2
  50/1 -> 68/2, in_range_Ib/1  "in_range_Ib"
  68/1 -> in_range_Iph/1  "in_range_Iph"
  25/1 -> Ia_im_CT1/1, 39/1
  70/1 -> 71/2, 69/2
  I30_re_CT2_sec/1 -> I0_2/1(Re), 74/1
  I30_im_CT2_sec/1 -> I0_2/2(Im), 75/1
  I30_re_CT1_sec/1 -> I0_1/1(Re), 72/1
  I30_im_CT1_sec/1 -> I0_1/2(Im), 73/1
  31/1 -> Ia_im_CT2/1, 39/2
  73/1 -> 71/1, 80/1
  72/1 -> 79/1, 69/1
  71/1 -> I0_im_CT1/1  "K_dop"
  69/1 -> I0_re_CT1/1  "K_dop"
  77/1 -> 78/2, 76/2
  78/1 -> I0_im/1  "K_dop"
  76/1 -> I0_re/1  "K_dop"
  79/1 -> 76/1  "Ic_re"
  80/1 -> 78/1  "Ic_im"
  81/1 -> I0_re_CT2/1  "K_dop"
  83/1 -> I0_im_CT2/1  "K_dop"
  82/1 -> 83/2, 81/2
  74/1 -> 81/1, 79/2
  75/1 -> 83/1, 80/2
  84/1 -> in_range_I0/1  "in_range_I0"
  85/1 -> 84/3  "in_range_Ic"
  I0_1/1(Module) -> 87/1
  I0_2/1(Module) -> 88/1
  87/1 -> 89/1
  88/1 -> 90/1
  86/1 -> 85/3  "in_range_Ic"
  91/1 -> 92/1
  92/1 -> 85/1
  7/1 -> in_range_Ib_CT1/1, 93/2, 53/1, 44/1  "in_range_Ib_CT1"
  89/1 -> in_range_I0_CT1/1, 86/1, 91/1  "in_range_I0_CT1"
  9/1 -> in_range_Ia_CT1/1, 93/1, 52/1, 14/1  "in_range_Ia_CT1"
  8/1 -> 54/1, 45/1, in_range_Ic_CT1/1, 93/3  "in_range_Ic_CT1"
  93/1 -> in_range_Iph_CT1/1  "in_range_Iph_CT1"
  12/1 -> 94/3, in_range_Ic_CT2/1, 54/3, 45/2  "in_range_Ic_CT2"
  94/1 -> in_range_Iph_CT2/1  "in_range_Iph_CT2"
  10/1 -> 94/1, in_range_Ia_CT2/1, 52/3, 14/2  "in_range_Ia_CT2"
  90/1 -> in_range_I0_CT2/1, 86/3, 91/2  "in_range_I0_CT2"
  11/1 -> 94/2, in_range_Ib_CT2/1, 53/3, 44/2  "in_range_Ib_CT2"

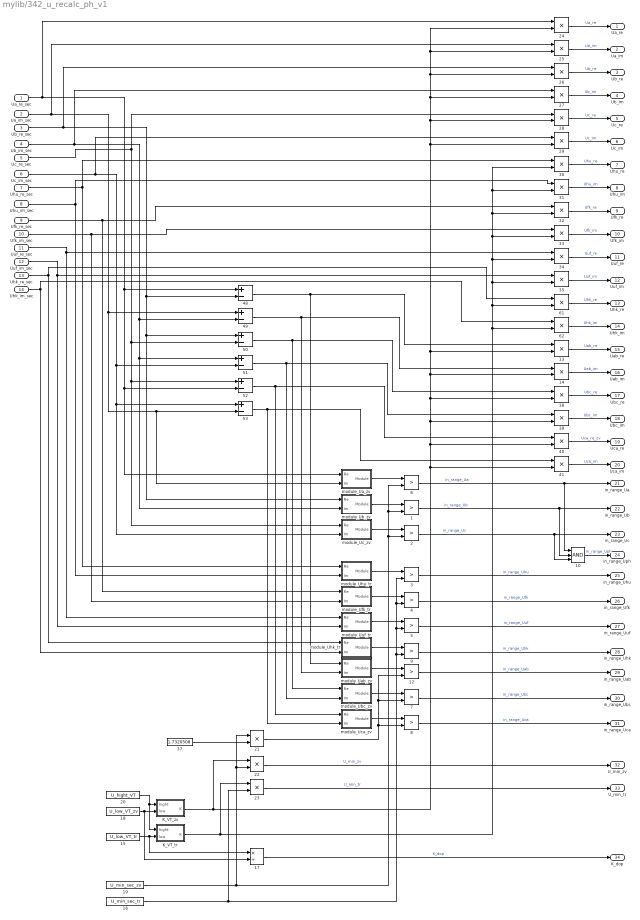
== system mylib/342_u_recalc_ph_v1 ==
  Ua_re_sec : Inport
  Ua_im_sec : Inport  Port=2
  Ub_re_sec : Inport  Port=3
  Ub_im_sec : Inport  Port=4
  Uc_re_sec : Inport  Port=5
  Uc_im_sec : Inport  Port=6
  Uhu_re_sec : Inport  Port=7
  Uhu_im_sec : Inport  Port=8
  Ufk_re_sec : Inport  Port=9
  Ufk_im_sec : Inport  Port=10
  Uuf_re_sec : Inport  Port=11
  Uuf_im_sec : Inport  Port=12
  Uhk_re_sec : Inport  Port=13
  Uhk_im_sec : Inport  Port=14
  {1..9,12} (10 alike) : RelationalOperator  Operator=>  OutDataTypeStr=boolean  RndMeth=Nearest
  10 : Logic  Inputs=3  AllPortsSameDT=off  OutDataTypeStr=boolean
  {13..14,21..35,38..41,61..62} (23 alike) : Product  Inputs=**  RndMeth=Zero  SaturateOnIntegerOverflow=on
  15 : Constant  Value=U_low_VT_tr
  16 : Constant  Value=U_min_sec_tr
  17 : Product  Inputs=*/  RndMeth=Zero  SaturateOnIntegerOverflow=on
  18 : Constant  Value=U_low_VT_zv
  19 : Constant  Value=U_min_sec_zv
  20 : Constant  Value=U_hight_VT
  37 : Constant  Value=1.7320508
  {48..53} (6 alike) : Sum  Inputs=+-
  K_VT_tr : Subsystem
  K_VT_zv : Subsystem
  module_Ua_zv : Subsystem
  module_Uab_zv : Subsystem
  module_Ub_zv : Subsystem
  module_Ubc_zv : Subsystem
  module_Uc_zv : Subsystem
  module_Uca_zv : Subsystem
  module_Ufk_tr : Subsystem
  module_Uhk_tr : Subsystem
  module_Uhu_tr : Subsystem
  module_Uuf_tr : Subsystem
  Ua_re : Outport
  Ua_im : Outport  Port=2
  Ub_re : Outport  Port=3
  Ub_im : Outport  Port=4
  Uc_re : Outport  Port=5
  Uc_im : Outport  Port=6
  Uhu_re : Outport  Port=7
  Uhu_im : Outport  Port=8
  Ufk_re : Outport  Port=9
  Ufk_im : Outport  Port=10
  Uuf_re : Outport  Port=11
  Uuf_im : Outport  Port=12
  Uhk_re : Outport  Port=13
  Uhk_im : Outport  Port=14
  Uab_re : Outport  Port=15
  Uab_im : Outport  Port=16
  Ubc_re : Outport  Port=17
  Ubc_im : Outport  Port=18
  Uca_re : Outport  Port=19
  Uca_im : Outport  Port=20
  in_range_Ua : Outport  Port=21
  in_range_Ub : Outport  Port=22
  in_range_Uc : Outport  Port=23
  in_range_Uph : Outport  Port=24
  in_range_Uhu : Outport  Port=25
  in_range_Ufk : Outport  Port=26
  in_range_Uuf : Outport  Port=27
  in_range_Uhk : Outport  Port=28
  in_range_Uab : Outport  Port=29
  in_range_Ubc : Outport  Port=30
  in_range_Uca : Outport  Port=31
  U_min_zv : Outport  Port=32
  U_min_tr : Outport  Port=33
  K_dop : Outport  Port=34
  wires:
  module_Ub_zv/1(Module) -> 1/1
  module_Ufk_tr/1(Module) -> 4/1
  module_Uuf_tr/1(Module) -> 5/1
  module_Uc_zv/1(Module) -> 2/1
  module_Ua_zv/1(Module) -> 6/1
  Ua_re_sec/1 -> 48/1, module_Ua_zv/1(Re), 52/2, 24/1
  Ufk_im_sec/1 -> 33/1, module_Ufk_tr/2(Im)
  Ub_im_sec/1 -> 49/2, 51/1, module_Ub_zv/2(Im), 27/1
  Uhu_re_sec/1 -> module_Uhu_tr/1(Re), 30/1
  Uhu_im_sec/1 -> module_Uhu_tr/2(Im), 31/1
  Uuf_re_sec/1 -> 34/1, module_Uuf_tr/1(Re)
  Uuf_im_sec/1 -> 35/1, module_Uuf_tr/2(Im)
  Uc_re_sec/1 -> 52/1, module_Uc_zv/1(Re), 50/2, 28/1
  20/1 -> K_VT_tr/1(hight), K_VT_zv/1(hight)
  18/1 -> 17/2, K_VT_zv/2(low)
  15/1 -> K_VT_tr/2(low), 17/1
  module_Uhu_tr/1(Module) -> 3/1
  Ua_im_sec/1 -> module_Ua_zv/2(Im), 53/2, 49/1, 25/1
  19/1 -> 2/2, 1/2, 6/2, 21/1, 22/2
  37/1 -> 21/2
  21/1 -> 8/2, 7/2, 12/2
  17/1 -> K_dop/1  "K_dop"
  module_Ubc_zv/1(Module) -> 7/1
  module_Uca_zv/1(Module) -> 8/1
  module_Uab_zv/1(Module) -> 12/1
  24/1 -> Ua_re/1  "Ua_re"
  25/1 -> Ua_im/1  "Ua_im"
  26/1 -> Ub_re/1  "Ub_re"
  27/1 -> Ub_im/1  "Ub_im"
  28/1 -> Uc_re/1  "Uc_re"
  29/1 -> Uc_im/1  "Uc_im"
  30/1 -> Uhu_re/1  "Uhu_re"
  31/1 -> Uhu_im/1  "Uhu_im"
  32/1 -> Ufk_re/1  "Ufk_re"
  33/1 -> Ufk_im/1  "Ufk_im"
  34/1 -> Uuf_re/1  "Uuf_re"
  35/1 -> Uuf_im/1  "Uuf_im"
  13/1 -> Uab_re/1  "Uab_re"
  14/1 -> Uab_im/1  "Uab_im"
  38/1 -> Ubc_re/1  "Ubc_re"
  39/1 -> Ubc_im/1  "Ubc_im"
  40/1 -> Uca_re/1  "Uca_re_zv"
  41/1 -> Uca_im/1  "Uca_im"
  6/1 -> 10/1, in_range_Ua/1  "in_range_Ua"
  1/1 -> 10/2, in_range_Ub/1  "in_range_Ub"
  2/1 -> 10/3, in_range_Uc/1  "in_range_Uc"
  3/1 -> in_range_Uhu/1  "in_range_Uhu"
  4/1 -> in_range_Ufk/1  "in_range_Ufk"
  5/1 -> in_range_Uuf/1  "in_range_Uuf"
  12/1 -> in_range_Uab/1  "in_range_Uab"
  7/1 -> in_range_Ubc/1  "in_range_Ubc"
  8/1 -> in_range_Uca/1  "in_range_Uca"
  48/1 -> module_Uab_zv/1(Re), 13/1
  49/1 -> module_Uab_zv/2(Im), 14/1
  50/1 -> module_Ubc_zv/1(Re), 38/1
  51/1 -> module_Ubc_zv/2(Im), 39/1
  52/1 -> module_Uca_zv/1(Re), 40/1
  53/1 -> module_Uca_zv/2(Im), 41/1
  Ub_re_sec/1 -> module_Ub_zv/1(Re), 50/1, 48/2, 26/1
  Uc_im_sec/1 -> 53/1, module_Uc_zv/2(Im), 51/2, 29/1
  Ufk_re_sec/1 -> module_Ufk_tr/1(Re), 32/1
  16/1 -> 9/2, 5/2, 4/2, 3/2, 23/2
  22/1 -> U_min_zv/1  "U_min_zv"
  23/1 -> U_min_tr/1  "U_min_tr"
  K_VT_zv/1(K) -> 29/2, 28/2, 27/2, 26/2, 25/2, 24/2, 13/2, 14/2, 38/2, 39/2, 40/2, 41/2, 22/1
  K_VT_tr/1(K) -> 62/2, 61/2, 35/2, 34/2, 33/2, 32/2, 31/2, 30/2, 23/1
  62/1 -> Uhk_im/1  "Uhk_im"
  61/1 -> Uhk_re/1  "Uhk_re"
  module_Uhk_tr/1(Module) -> 9/1
  9/1 -> in_range_Uhk/1  "in_range_Uhk"
  10/1 -> in_range_Uph/1  "in_range_Uph"
  Uhk_re_sec/1 -> module_Uhk_tr/1(Re), 61/1
  Uhk_im_sec/1 -> module_Uhk_tr/2(Im), 62/1

== system mylib/Inverse time-delay ==
  I : Inport
  ANSI Inverse time-delay : Subsystem
  ANSI Inverse time-delay inductive disk relay : Subsystem
  Add : Sum
  Constant : Constant  Value=IEC_N
  Constant1 : Constant  Value=ku_IEC
  Constant10 : Constant  Value=Au_ANSI
  Constant11 : Constant  Value=Bu_ANSI
  Constant12 : Constant  Value=Au_ANSI_idr
  Constant13 : Constant  Value=ANSI_N
  Constant14 : Constant  Value=Bu_ANSI_idr
  Constant15 : Constant  Value=ANSI_N_idr
  Constant16 : Constant  Value=Cu_ANSI_idr
  Constant17 : Constant  Value=IDR
  Constant18 : Constant  Value=0
  Constant19 : Constant  Value=0
  Constant2 : Constant  Value=au_IEC
  Constant20 : Constant  Value=Type_ITD
  Constant21 : Constant  Value=Cu_ANSI
  Constant3 : Constant  Value=Tb
  Constant5 : Constant  Value=ku_IEC_idr
  Constant6 : Constant  Value=au_IEC_idr
  Constant7 : Constant  Value=Ip
  Constant8 : Constant  Value=D
  Constant9 : Constant  Value=IEC_N_idr
  IEC Inverse time-delay : Subsystem
  IEC Inverse time-delay inductive disk relay : Subsystem
  Logical Operator : Logic  AllPortsSameDT=off  OutDataTypeStr=boolean
  Logical Operator1 : Logic  AllPortsSameDT=off  OutDataTypeStr=boolean
  Logical Operator4 : Logic  Operator=NOT  AllPortsSameDT=off  OutDataTypeStr=boolean
  Switch1 : Switch  Criteria=u2 > Threshold
  Switch2 : Switch  Criteria=u2 > Threshold
  Switch3 : Switch  Criteria=u2 > Threshold
  tp : Outport
  td : Outport  Port=2
  wires:
  IEC Inverse time-delay/1(td) -> Switch3/1
  Logical Operator4/1 -> Logical Operator1/1
  Constant8/1 -> ANSI Inverse time-delay/7(D), ANSI Inverse time-delay inductive disk relay/7(D)
  Constant6/1 -> IEC Inverse time-delay inductive disk relay/4(au_IEC_idr)
  Constant15/1 -> ANSI Inverse time-delay inductive disk relay/2(ANSI_N_idr)
  Constant16/1 -> ANSI Inverse time-delay inductive disk relay/5(Cu_ANSI_idr)
  Constant12/1 -> ANSI Inverse time-delay inductive disk relay/3(Au_ANSI_idr)
  ANSI Inverse time-delay inductive disk relay/1(td) -> Switch2/1
  Switch2/1 -> Add/2
  Constant/1 -> IEC Inverse time-delay/2(IEC_N)
  Logical Operator1/1 -> Switch2/2
  Constant17/1 -> Logical Operator/2, Logical Operator1/2
  Constant5/1 -> IEC Inverse time-delay inductive disk relay/3(ku_IEC_idr)
  I/1 -> IEC Inverse time-delay inductive disk relay/1(I), ANSI Inverse time-delay inductive disk relay/1(I), ANSI Inverse time-delay/1(I), IEC Inverse time-delay/1(I)
  Constant19/1 -> Switch1/3
  Logical Operator/1 -> Switch1/2
  Switch1/1 -> Add/1
  Constant7/1 -> ANSI Inverse time-delay inductive disk relay/6(Ip), ANSI Inverse time-delay/6(Ip), IEC Inverse time-delay inductive disk relay/5(Ip), IEC Inverse time-delay/5(Ip)
  Switch3/1 -> tp/1
  Constant20/1 -> Logical Operator4/1, Switch3/2, Logical Operator/1
  Constant18/1 -> Switch2/3
  Constant3/1 -> IEC Inverse time-delay inductive disk relay/6(Tb), IEC Inverse time-delay/6(Tb)
  Add/1 -> td/1
  Constant10/1 -> ANSI Inverse time-delay/3(Au_ANSI)
  Constant2/1 -> IEC Inverse time-delay/4(au_IEC)
  IEC Inverse time-delay inductive disk relay/1(td) -> Switch1/1
  Constant11/1 -> ANSI Inverse time-delay/4(Bu_ANSI)
  Constant1/1 -> IEC Inverse time-delay/3(ku_IEC)
  Constant13/1 -> ANSI Inverse time-delay/2(ANSI_N)
  Constant14/1 -> ANSI Inverse time-delay inductive disk relay/4(Bu_ANSI_idr)
  Constant9/1 -> IEC Inverse time-delay inductive disk relay/2(IEC_N_idr)
  Constant21/1 -> ANSI Inverse time-delay/5(Cu_ANSI)
  ANSI Inverse time-delay/1(td) -> Switch3/3

== system mylib/Max_ph_value ==
  Re1 : Inport
  Im1 : Inport  Port=2
  Re2 : Inport  Port=3
  Im2 : Inport  Port=4
  Re3 : Inport  Port=5
  Im3 : Inport  Port=6
  Im_1 : Switch  Criteria=u2 > Threshold
  Im_2 : Switch  Criteria=u2 > Threshold
  Max_1 : Switch  Criteria=u2 > Threshold
  Max_2 : Switch  Criteria=u2 > Threshold
  ORTOTOMODULE2 : $bdroot/ORTOTOMODULE  SystemSampleTime=-1  Latency=0  AutoFrameSizeCalculation=off
  ORTOTOMODULE3 : $bdroot/ORTOTOMODULE  SystemSampleTime=-1  Latency=0  AutoFrameSizeCalculation=off
  ORTOTOMODULE4 : $bdroot/ORTOTOMODULE  SystemSampleTime=-1  Latency=0  AutoFrameSizeCalculation=off
  Re_1 : Switch  Criteria=u2 > Threshold
  Re_2 : Switch  Criteria=u2 > Threshold
  Relational Operator : RelationalOperator  OutDataTypeStr=boolean  RndMeth=Simplest
  Relational Operator1 : RelationalOperator  OutDataTypeStr=boolean  RndMeth=Simplest
  MaxRe : Outport
  MaxIm : Outport  Port=2
  Max_Val : Outport  Port=3
  wires:
  Im1/1 -> ORTOTOMODULE2/2, Im_1/1
  Im3/1 -> ORTOTOMODULE4/2, Im_2/3
  Re2/1 -> ORTOTOMODULE3/1, Re_1/3
  Re1/1 -> ORTOTOMODULE2/1, Re_1/1
  Re3/1 -> Re_2/3, ORTOTOMODULE4/1
  Im2/1 -> Im_1/3, ORTOTOMODULE3/2
  ORTOTOMODULE2/1 -> Max_1/1, Relational Operator/1
  ORTOTOMODULE3/1 -> Relational Operator/2, Max_1/3
  Relational Operator/1 -> Max_1/2, Im_1/2, Re_1/2
  Relational Operator1/1 -> Max_2/2, Re_2/2, Im_2/2
  Max_1/1 -> Max_2/1, Relational Operator1/1
  ORTOTOMODULE4/1 -> Relational Operator1/2, Max_2/3
  Im_1/1 -> Im_2/1
  Re_1/1 -> Re_2/1
  Max_2/1 -> Max_Val/1
  Im_2/1 -> MaxIm/1
  Re_2/1 -> MaxRe/1

== system mylib/Min_ph_value ==
  Re1 : Inport
  Im1 : Inport  Port=2
  Re2 : Inport  Port=3
  Im2 : Inport  Port=4
  Re3 : Inport  Port=5
  Im3 : Inport  Port=6
  Im_1 : Switch  Criteria=u2 > Threshold
  Im_2 : Switch  Criteria=u2 > Threshold
  Min_1 : Switch  Criteria=u2 > Threshold
  Min_2 : Switch  Criteria=u2 > Threshold
  ORTOTOMODULE2 : $bdroot/ORTOTOMODULE  SystemSampleTime=-1  Latency=0  AutoFrameSizeCalculation=off
  ORTOTOMODULE3 : $bdroot/ORTOTOMODULE  SystemSampleTime=-1  Latency=0  AutoFrameSizeCalculation=off
  ORTOTOMODULE4 : $bdroot/ORTOTOMODULE  SystemSampleTime=-1  Latency=0  AutoFrameSizeCalculation=off
  Re_1 : Switch  Criteria=u2 > Threshold
  Re_2 : Switch  Criteria=u2 > Threshold
  Relational Operator : RelationalOperator  Operator=<=  OutDataTypeStr=boolean  RndMeth=Simplest
  Relational Operator1 : RelationalOperator  Operator=<=  OutDataTypeStr=boolean  RndMeth=Simplest
  MinRe : Outport
  MinIm : Outport  Port=2
  Min_Val : Outport  Port=3
  wires:
  Im1/1 -> ORTOTOMODULE2/2, Im_1/1
  Im3/1 -> ORTOTOMODULE4/2, Im_2/3
  Re2/1 -> ORTOTOMODULE3/1, Re_1/3
  Re1/1 -> ORTOTOMODULE2/1, Re_1/1
  Re3/1 -> Re_2/3, ORTOTOMODULE4/1
  Im2/1 -> Im_1/3, ORTOTOMODULE3/2
  ORTOTOMODULE2/1 -> Min_1/1, Relational Operator/1
  ORTOTOMODULE3/1 -> Relational Operator/2, Min_1/3
  Relational Operator/1 -> Min_1/2, Im_1/2, Re_1/2
  Relational Operator1/1 -> Min_2/2, Re_2/2, Im_2/2
  Min_1/1 -> Min_2/1, Relational Operator1/1
  ORTOTOMODULE4/1 -> Relational Operator1/2, Min_2/3
  Im_1/1 -> Im_2/1
  Re_1/1 -> Re_2/1
  Min_2/1 -> Min_Val/1
  Im_2/1 -> MinIm/1
  Re_2/1 -> MinRe/1

== system mylib/ORTOTOMODULE ==
  Re : Inport
  Im : Inport  Port=2
  1 : Product  Inputs=**
  2 : Sum
  3 : Product  Inputs=**
  4 : Sqrt  SaturateOnIntegerOverflow=on
  Module : Outport
  wires:
  3/1 -> 2/2
  1/1 -> 2/1
  Im/1 -> 3/1, 3/2
  4/1 -> Module/1
  2/1 -> 4/1
  Re/1 -> 1/2, 1/1

== system mylib/RS ==
  S : Inport
  R : Inport  Port=2
  12 : Logic  AllPortsSameDT=off  OutDataTypeStr=boolean
  13 : Logic  Operator=NOT  AllPortsSameDT=off  OutDataTypeStr=boolean
  14 : Memory
  15 : Logic  Operator=OR  AllPortsSameDT=off  OutDataTypeStr=boolean
  Q : Outport
  wires:
  13/1 -> 12/2
  S/1 -> 15/2
  R/1 -> 13/1
  15/1 -> 12/1
  12/1 -> Q/1, 14/1
  14/1 -> 15/1

== system mylib/R_TRIG ==
  CLK : Inport
  26 : Logic  AllPortsSameDT=off  OutDataTypeStr=boolean
  27 : Logic  Operator=NOT  AllPortsSameDT=off  OutDataTypeStr=boolean
  Memory : Memory
  Q : Outport
  wires:
  27/1 -> 26/2
  Memory/1 -> 27/1
  CLK/1 -> Memory/1, 26/1
  26/1 -> Q/1

== system mylib/SR ==
  S : Inport
  R : Inport  Port=2
  12 : Logic  AllPortsSameDT=off  OutDataTypeStr=boolean
  13 : Logic  Operator=NOT  AllPortsSameDT=off  OutDataTypeStr=boolean
  14 : Memory
  15 : Logic  Operator=OR  AllPortsSameDT=off  OutDataTypeStr=boolean
  Q : Outport
  wires:
  R/1 -> 13/1
  S/1 -> 15/1
  13/1 -> 12/2
  14/1 -> 12/1
  15/1 -> 14/1, Q/1
  12/1 -> 15/2

== system mylib/delta_calc ==
  In1_re : Inport
  In1_im : Inport  Port=2
  In2_re : Inport  Port=3
  In2_im : Inport  Port=4
  1 : RelationalOperator  Operator=>  OutDataTypeStr=boolean  RndMeth=Simplest
  {4..6,10,12..13} (6 alike) : Product  Inputs=**
  11 : Sum
  {8..9,14..15} (4 alike) : Sum  Inputs=+-
  2 : Sum
  3 : Switch  Criteria=u2 > Threshold
  7 : Sum
  Acos : Trigonometry  Operator=acos
  Constant : Constant  Value=2
  Constant1 : Constant  Value=-1
  Constant2 : Constant
  Constant3 : Constant  Value=0.5
  Cos : Trigonometry  Operator=cos
  Sin : Trigonometry
  in1_to_pu : $bdroot/vect_to_pu  SystemSampleTime=-1  Latency=0  AutoFrameSizeCalculation=off
  in2_to_pu : $bdroot/vect_to_pu  SystemSampleTime=-1  Latency=0  AutoFrameSizeCalculation=off
  arg : Outport
  re : Outport  Port=2
  im : Outport  Port=3
  wires:
  In2_re/1 -> in2_to_pu/1
  In2_im/1 -> in2_to_pu/2
  In1_re/1 -> in1_to_pu/1
  In1_im/1 -> in1_to_pu/2
  Cos/1 -> re/1
  Sin/1 -> im/1
  3/1 -> arg/1, Sin/1, Cos/1
  Acos/1 -> 5/1, 3/3
  5/1 -> 3/1
  1/1 -> 3/2
  2/1 -> 1/1
  Constant/1 -> 1/2
  4/1 -> 2/1
  6/1 -> 2/2
  7/1 -> 6/1, 6/2
  8/1 -> 4/1, 4/2
  in2_to_pu/2 -> 15/2, 7/2
  in1_to_pu/2 -> 15/1, 8/1
  in2_to_pu/1 -> 14/2, 8/2
  Constant1/1 -> 5/2
  9/1 -> Acos/1
  Constant2/1 -> 9/1
  10/1 -> 9/2
  11/1 -> 10/1
  Constant3/1 -> 10/2
  12/1 -> 11/1
  13/1 -> 11/2
  14/1 -> 12/2, 12/1
  15/1 -> 13/2, 13/1
  in1_to_pu/1 -> 14/1, 7/1

== system mylib/derivative ==
  A : Inport
  1 : Constant  Value=0.3333333
  10 : Product  Inputs=*/  RndMeth=Zero  SaturateOnIntegerOverflow=on
  11 : Abs
  12 : Sum  Inputs=+++
  13 : Product
  14 : Sum  Inputs=+-
  6 : Switch  Criteria=u2 > Threshold
  7 : RelationalOperator  Operator===  OutDataTypeStr=boolean  RndMeth=Simplest
  8 : Constant  Value=0
  9 : Constant  Value=0.0000001
  fifo2 : Subsystem
  Y : Outport
  Y_abs : Outport  Port=2
  wires:
  A/1 -> fifo2/1(y)
  6/1 -> 10/2
  11/1 -> 10/1, Y_abs/1
  10/1 -> Y/1
  7/1 -> 6/2
  8/1 -> 7/2
  fifo2/6(y5) -> 12/1
  fifo2/7(y6) -> 12/2
  fifo2/8(y7) -> 12/3
  12/1 -> 13/1
  1/1 -> 13/2
  9/1 -> 6/1
  13/1 -> 14/2, 7/1, 6/3
  14/1 -> 11/1
  fifo2/1(y0) -> 14/1

== system mylib/in_jmp ==
  jmp_in_zone : Inport
  in : Inport  Port=2
  jmp : Inport  Port=3
  1 : Switch  Criteria=u2 > Threshold
  10 : Logic  AllPortsSameDT=off  OutDataTypeStr=boolean
  11 : Logic  Operator=NOT  AllPortsSameDT=off  OutDataTypeStr=boolean
  12 : Memory
  3 : Logic  AllPortsSameDT=off  OutDataTypeStr=boolean
  RS : $bdroot/RS  SystemSampleTime=-1  Latency=0  AutoFrameSizeCalculation=off
  R_TRIG : $bdroot/R_TRIG  SystemSampleTime=-1  Latency=0  AutoFrameSizeCalculation=off
  T1 : powerlib_meascontrol/Logic/On Delay  DelayType=Off delay  delay=T_reset  ic=1  Ts=0
  T2 : powerlib_meascontrol/Logic/On Delay  DelayType=On delay  delay=T_reset  ic=1  Ts=0
  Y : Outport
  wires:
  RS/1 -> 12/1, Y/1
  in/1 -> 11/1, R_TRIG/1, 1/3
  R_TRIG/1 -> 1/1
  jmp_in_zone/1 -> 1/2
  11/1 -> 10/2
  10/1 -> T2/1
  T1/1 -> 3/2
  1/1 -> 3/1
  jmp/1 -> T1/1
  12/1 -> 10/1
  T2/1 -> RS/2
  3/1 -> RS/1

== system mylib/orto_DIV_orto ==
  F1re : Inport
  F1im : Inport  Port=2
  F2re : Inport  Port=3
  F2im : Inport  Port=4
  1 : Sum  Inputs=+-
  {2..5,7..8} (6 alike) : Product
  6 : Sum
  9 : Sum
  Constant : Constant  Value=0.0000000001
  Divide : Product  Inputs=*/
  Divide1 : Product  Inputs=*/
  Relational Operator : RelationalOperator  Operator=<  OutDataTypeStr=boolean  RndMeth=Simplest
  Switch : Switch  Criteria=u2 > Threshold
  Fre : Outport
  Fim : Outport  Port=2
  wires:
  4/1 -> 1/1
  5/1 -> 1/2
  7/1 -> 9/1
  8/1 -> 9/2
  3/1 -> 6/2
  2/1 -> 6/1
  6/1 -> Divide/1
  Divide/1 -> Fre/1
  F1re/1 -> 5/1, 2/1
  9/1 -> Relational Operator/1, Switch/3
  Constant/1 -> Switch/1, Relational Operator/2
  Relational Operator/1 -> Switch/2
  F2re/1 -> 2/2, 4/2, 7/2, 7/1
  F2im/1 -> 3/2, 5/2, 8/2, 8/1
  Switch/1 -> Divide1/2, Divide/2
  1/1 -> Divide1/1
  F1im/1 -> 4/1, 3/1
  Divide1/1 -> Fim/1

== system mylib/orto_MUL_orto ==
  F1re : Inport
  F1im : Inport  Port=2
  F2re : Inport  Port=3
  F2im : Inport  Port=4
  1 : Sum  Inputs=+-
  {2..5} (4 alike) : Product
  6 : Sum
  Fre : Outport
  Fim : Outport  Port=2
  wires:
  F2re/1 -> 4/2, 2/2
  F1im/1 -> 3/1, 4/1
  F2im/1 -> 3/2, 5/2
  5/1 -> 6/2
  4/1 -> 6/1
  3/1 -> 1/2
  2/1 -> 1/1
  6/1 -> Fim/1
  1/1 -> Fre/1
  F1re/1 -> 2/1, 5/1

== system mylib/orto_to_arg ==
  re : Inport
  im : Inport  Port=2
  1 : Sum
  11 : Product  Inputs=*/  RndMeth=Zero  SaturateOnIntegerOverflow=on
  154 : Constant  Value=-1
  2 : Product
  3 : Switch  Criteria=u2 > Threshold
  4 : Sqrt  SaturateOnIntegerOverflow=on
  5 : Trigonometry  Operator=acos
  6 : Product
  7 : RelationalOperator  Operator=>  OutDataTypeStr=boolean  RndMeth=Simplest
  8 : Constant  Value=0
  9 : Product
  arg : Outport
  wires:
  4/1 -> 11/2
  11/1 -> 5/1
  2/1 -> 1/1
  6/1 -> 1/2
  1/1 -> 4/1
  5/1 -> 9/1, 3/1
  154/1 -> 9/2
  7/1 -> 3/2
  9/1 -> 3/3
  8/1 -> 7/2
  re/1 -> 2/1, 11/1, 2/2
  im/1 -> 6/1, 6/2, 7/1
  3/1 -> arg/1

== system mylib/out3 ==
  in : Inport
  1 : Logic  Operator=OR  AllPortsSameDT=off  OutDataTypeStr=boolean
  2 : powerlib_meascontrol/Logic/Monostable  EdgeDetect=Rising  PulseDuration=T_out  ic=0  Ts=0
      settings: SourceProductBaseCode=PS
  R_TRIG : $bdroot/R_TRIG  SystemSampleTime=-1  Latency=0  AutoFrameSizeCalculation=off
  out : Outport
  wires:
  2/1 -> 1/2
  1/1 -> out/1
  R_TRIG/1 -> 1/1
  in/1 -> R_TRIG/1, 2/1
